simulink model "mdlWiW2025"  (R2024b)
settings: Solver=FixedStepAuto  StartTime=0.0  StopTime=p.simTime  FixedStep=5e-5  MaxStep=1e-4  RelTol=1e-3
values from neighbouring files (symbols this model uses):
  a0_WT_Act_DC_Inv = a0    [RunTestCasesWiW2025.m]    (also in mainWiW2025.m)
  A_WT_Act_DC_Inv = A    [RunTestCasesWiW2025.m]    (also in mainWiW2025.m)
  B_WT_Act_DC_Inv = Bu    [RunTestCasesWiW2025.m]    (also in mainWiW2025.m)
  Bd_WT_Act_DC_Inv = Bd    [RunTestCasesWiW2025.m]    (also in mainWiW2025.m)
  Cag = p.LTIAngleGen.Cz(1,:)    [RunTestCasesWiW2025.m]    (also in mainWiW2025.m)
  Cd_WT_Act_DC_Inv = Cd    [RunTestCasesWiW2025.m]    (also in mainWiW2025.m)
  Cu_WT_Act_DC_Inv = Cu    [RunTestCasesWiW2025.m]    (also in mainWiW2025.m)
  Cx_WT_Act_DC_Inv = Cx    [RunTestCasesWiW2025.m]    (also in mainWiW2025.m)
  p = loadTestCasesWiW2025(p)    [RunTestCasesWiW2025.m]    (also in mainWiW2025.m)
  parWT_Init = calcInitWTV2(parWT_Init,parWT,PrefInv0,v_wind_pu0)    [RunTestCasesWiW2025.m]    (also in mainWiW2025.m)
  xInit_WT_Act_DC_Inv = x0    [RunTestCasesWiW2025.m]    (also in mainWiW2025.m)
undefined symbols (not defined in the file or in its folder): DiscIntNeverNeededParam, height, KuDC, parDC, parInvLinMdl, parSim, parWT
libraries: simulink x14, simulink_extras x6
settings Model: Creator=jb  LastModifiedBy=jb

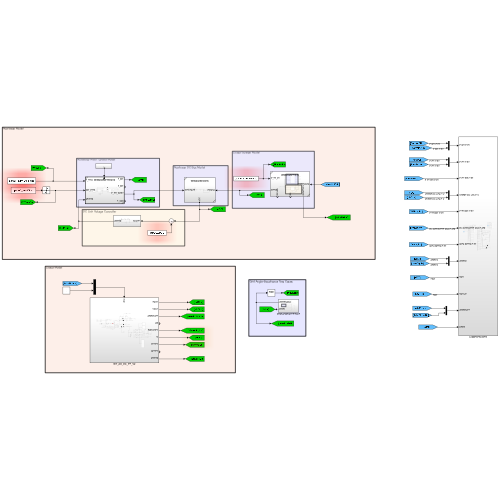
[thumbnail: Simulink's stored preview of the top-level diagram]
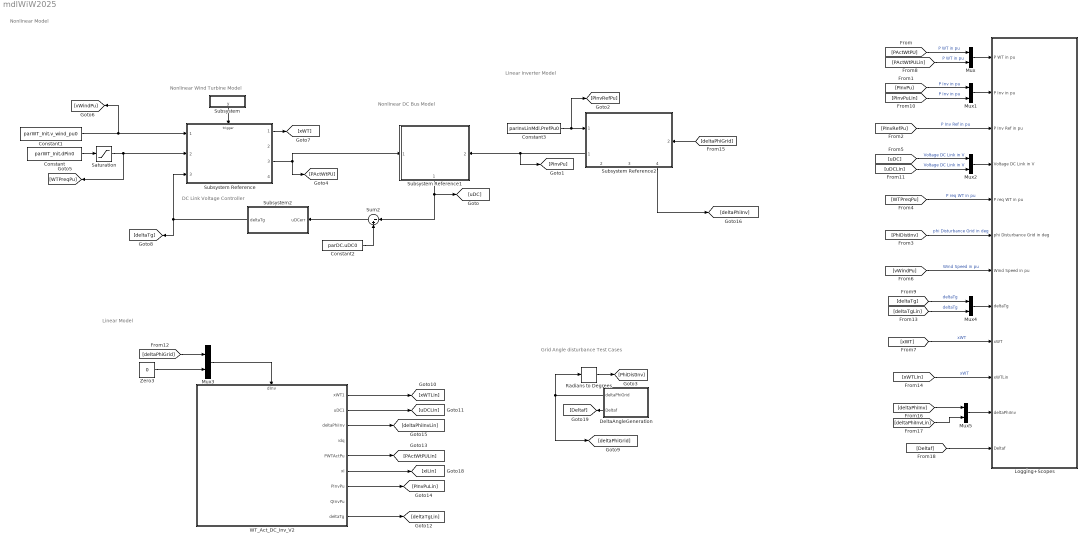
== system mdlWiW2025 ==
  note: Linear Model
  note: Nonlinear Model
  note: Grid Angle disturbance Test Cases
  note: Linear Inverter Model
  note: Nonlinear DC Bus Model
  note: Nonlinear Wind Turbine Model
  note: DC Link Voltage Controller
  Constant : Constant  Value=parWT_Init.dPin0
  Constant1 : Constant  Value=parWT_Init.v_wind_pu0
  Constant2 : Constant  Value=parDC.uDC0
  Constant3 : Constant  Value=parInvLinMdl.PrefPu0
  DeltaAngleGeneration : Subsystem
  Logging+Scopes : Subsystem
  Mux{,1..5} (6 alike) : Mux  Inputs=2
  Radians to Degrees : simulink_extras/Transformations/Radians to Degrees
  Saturation : Saturate  UpperLimit=1  LowerLimit=0
  Subsystem : Subsystem
      settings: PortSchema="{\"entries\":[{\"content\":{\"sides\":[{\"content\":{},\"type\":\"ConnectorPlacement.EquallySpacedRectSide\",\"uuid\":\"face2676-c510-409b-bee4-6c32a14faacb\"},{\"content\":{\"side\":\"RIGHT\"},\"type\":\"ConnectorPlacement.EquallySpacedRectSide\",\"uuid\":\"830bd05e-6053-45eb-9a2c-0b303f31509f\"},{\"content\":{\"side\":\"TOP\"},\"type\":\"ConnectorPlacement.EquallySpacedRectSide\",\"uuid\":\"8cce3491-981c-4252-b01c-3725d9c0f3f5\"},{\"content\":{\"connectorIds\":[\"Out1\"],\"side\":\"BOTTOM\"},\"type\":\"ConnectorPlacement.EquallySpacedRectSide\",\"uuid\":\"0505e35c-7957-4f95-90e0-2f2f2a48fa2e\"}]},\"type\":\"ConnectorPlacement.EquallySpacedConnector\",\"uuid\":\"a006b626-9c6b-4b47-b9fe-26644a837cf6\"}],\"packageUris\":[\"http://schema.mathworks.com/mf0/Connector/R2020b\"],\"version\":\"1.0\"}"
  Subsystem Reference : Subsystem  ReferencedSubsystem=WiW2025WTSubV2
  Subsystem Reference1 : Subsystem  ReferencedSubsystem=WiW2025DCSub
      settings: PortSchema="{\"entries\":[{\"content\":{\"sides\":[{\"content\":{\"connectorIds\":[\"In1\"]},\"type\":\"ConnectorPlacement.EquallySpacedRectSide\",\"uuid\":\"af152640-0aea-4f78-87a2-77a2b6d9cc3d\"},{\"content\":{\"connectorIds\":[\"In2\"],\"side\":\"RIGHT\"},\"type\":\"ConnectorPlacement.EquallySpacedRectSide\",\"uuid\":\"c02e3cac-108b-419e-ba46-7a5e2003643a\"},{\"content\":{\"side\":\"TOP\"},\"type\":\"ConnectorPlacement.EquallySpacedRectSide\",\"uuid\":\"91b439c3-63cc-4837-83b1-e86f1ef1a4a8\"},{\"content\":{\"connectorIds\":[\"Out1\"],\"side\":\"BOTTOM\"},\"type\":\"ConnectorPlacement.EquallySpacedRectSide\",\"uuid\":\"d1b53956-1662-4620-938c-5b6d0f97b7d8\"}]},\"type\":\"ConnectorPlacement.EquallySpacedConnector\",\"uuid\":\"de17c35b-190b-4b93-b08c-74ec9942f8f8\"}],\"packageUris\":[\"http://schema.mathworks.com/mf0/Connector/R2020b\"],\"version\":\"1.0\"}"
  Subsystem Reference2 : Subsystem  ReferencedSubsystem=WIW2025InvSub
      settings: PortSchema="{\"entries\":[{\"content\":{\"sides\":[{\"content\":{\"connectorIds\":[\"In1\",\"Out1\"]},\"type\":\"ConnectorPlacement.EquallySpacedRectSide\",\"uuid\":\"cb46f29d-b99f-4ee2-b312-1d4d79ed2caa\"},{\"content\":{\"connectorIds\":[\"In2\"],\"side\":\"RIGHT\"},\"type\":\"ConnectorPlacement.EquallySpacedRectSide\",\"uuid\":\"26f24ffb-094e-4bd5-ac8a-0db6a0458604\"},{\"content\":{\"side\":\"TOP\"},\"type\":\"ConnectorPlacement.EquallySpacedRectSide\",\"uuid\":\"c74ec33e-f362-4649-ae41-595cc258bb20\"},{\"content\":{\"connectorIds\":[\"Out2\",\"Out3\",\"Out4\"],\"side\":\"BOTTOM\"},\"type\":\"ConnectorPlacement.EquallySpacedRectSide\",\"uuid\":\"007ad1bf-c446-4ada-ae47-7c61a598a283\"}]},\"type\":\"ConnectorPlacement.EquallySpacedConnector\",\"uuid\":\"d7ac4c6f-570b-43ee-bac2-909fe494d4ed\"}],\"packageUris\":[\"http://schema.mathworks.com/mf0/Connector/R2020b\"],\"version\":\"1.0\"}"
  Subsystem2 : Subsystem
  Sum2 : Sum  Inputs=|-+
  WT_Act_DC_Inv_V2 : Subsystem
      settings: PortSchema="{\"entries\":[{\"content\":{\"sides\":[{\"content\":{},\"type\":\"ConnectorPlacement.EquallySpacedRectSide\",\"uuid\":\"d496482a-58bf-4391-9899-88596b85405c\"},{\"content\":{\"connectorIds\":[\"Out1\",\"Out2\",\"Out3\",\"Out4\",\"Out5\",\"Out6\",\"Out7\",\"Out8\",\"Out9\"],\"side\":\"RIGHT\"},\"type\":\"ConnectorPlacement.EquallySpacedRectSide\",\"uuid\":\"a3404192-e98c-40d4-9c55-e554f3dcbbe4\"},{\"content\":{\"connectorIds\":[\"In1\"],\"side\":\"TOP\"},\"type\":\"ConnectorPlacement.EquallySpacedRectSide\",\"uuid\":\"9344e298-d4d2-4a1e-a643-46297d368621\"}]},\"type\":\"ConnectorPlacement.EquallySpacedConnector\",\"uuid\":\"f7f68960-7837-437b-8e14-1803fee5da4e\"}],\"packageUris\":[\"http://schema.mathworks.com/mf0/Connector/R2020b\"],\"version\":\"1.0\"}"
  Zero3 : Constant  Value=0  OutDataTypeStr=Inherit: Inherit via back propagation
  wires:
  Constant/1 -> Saturation/1
  DeltaAngleGeneration/1(deltaPhiGrid) -> [deltaPhiGrid], Radians to Degrees/1
  Constant1/1 -> Subsystem Reference/1, [vWindPu]
  Radians to Degrees/1 -> [PhiDistInv]
  Saturation/1 -> Subsystem Reference/2, [WTPreqPu]
  Subsystem Reference/1 -> [xWT]
  Subsystem/1(y) -> Subsystem Reference/Trigger
  Sum2/1 -> Subsystem2/1(uDCerr)
  Constant2/1 -> Sum2/2
  Subsystem Reference1/1 -> Sum2/1, [uDC]
  Subsystem Reference/3 -> Subsystem Reference1/1, [PActWtPU]
  Subsystem2/1(deltaTg) -> [deltaTg], Subsystem Reference/3
  Constant3/1 -> [PInvRefPu], Subsystem Reference2/1
  Subsystem Reference2/1 -> [PInvPu], Subsystem Reference1/2
  [deltaPhiGrid] -> Mux3/1
  Mux3/1 -> WT_Act_DC_Inv_V2/1(dInv)
  Zero3/1 -> Mux3/2
  WT_Act_DC_Inv_V2/1(xWT1) -> [xWTLin]
  WT_Act_DC_Inv_V2/2(uDC1) -> [uDCLin]
  WT_Act_DC_Inv_V2/9(deltaTg) -> [deltaTgLin]
  WT_Act_DC_Inv_V2/7(PInvPu) -> [PInvPuLin]
  [PActWtPU] -> Mux/1  "P WT in pu"
  [PInvPu] -> Mux1/1  "P Inv in pu"
  [PInvRefPu] -> Logging+Scopes/3(P Inv Ref in pu)  "P Inv Ref in pu"
  [uDC] -> Mux2/1  "Voltage DC Link in V"
  [deltaTg] -> Mux4/1  "deltaTg"
  [xWT] -> Logging+Scopes/9(xWT)  "xWT"
  [vWindPu] -> Logging+Scopes/7(Wind Speed in pu)  "Wind Speed in pu"
  [PhiDistInv] -> Logging+Scopes/6(phi Disturbance Grid in deg)  "phi Disturbance Grid in deg"
  [WTPreqPu] -> Logging+Scopes/5(P req WT in pu)  "P req WT in pu"
  Mux2/1 -> Logging+Scopes/4(Voltage DC Link in V)
  Mux1/1 -> Logging+Scopes/2(P Inv in pu)
  Mux/1 -> Logging+Scopes/1(P WT in pu)
  [PActWtPULin] -> Mux/2  "P WT in pu"
  [PInvPuLin] -> Mux1/2  "P Inv in pu"
  [uDCLin] -> Mux2/2  "Voltage DC Link in V"
  [deltaTgLin] -> Mux4/2  "deltaTg"
  Mux4/1 -> Logging+Scopes/8(deltaTg)
  [xWTLin] -> Logging+Scopes/10(xWTLin)  "xWT"
  [deltaPhiGrid] -> Subsystem Reference2/2
  WT_Act_DC_Inv_V2/5(PWTActPu) -> [PActWtPULin]
  WT_Act_DC_Inv_V2/3(deltaPhiInv) -> [deltaPhiInvLin]
  Subsystem Reference2/4 -> [deltaPhiInv]
  Mux5/1 -> Logging+Scopes/11(deltaPhiInv)
  [deltaPhiInv] -> Mux5/1
  [deltaPhiInvLin] -> Mux5/2
  WT_Act_DC_Inv_V2/6(xI) -> [xILin]
  DeltaAngleGeneration/2(Deltaf) -> [Deltaf]
  [Deltaf] -> Logging+Scopes/12(Deltaf)

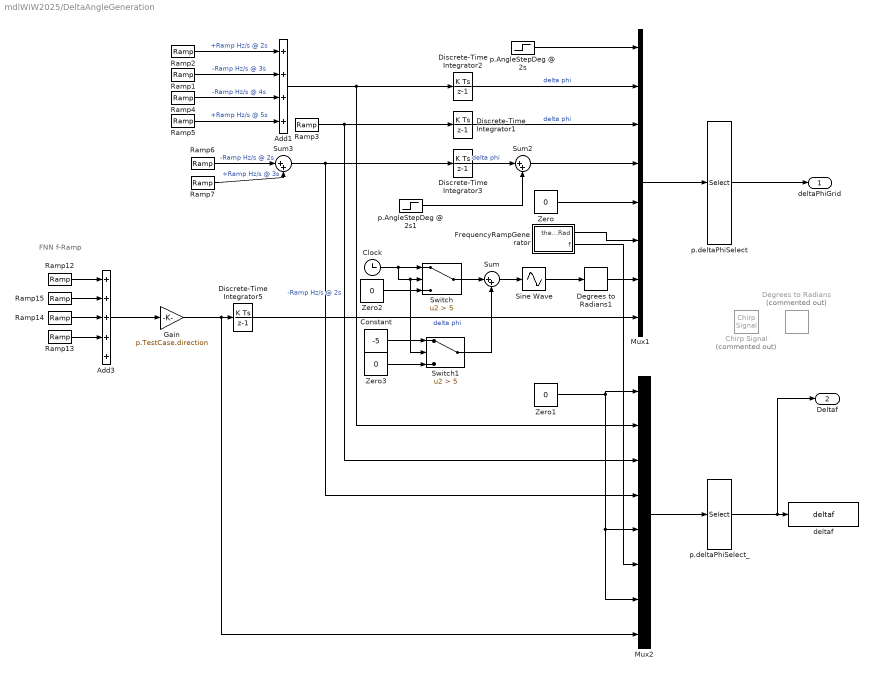
== system mdlWiW2025/DeltaAngleGeneration ==
  note: FNN f-Ramp
  Add1 : Sum  Inputs=++++
  Add3 : Sum  Inputs=+++++
  Chirp Signal : simulink/Sources/Chirp Signal  Commented=on  f1=0.1  T=80  f2=5
  Clock : Clock
  Constant : Constant  Value=-5
  Degrees to Radians : simulink_extras/Transformations/Degrees to Radians  Commented=on
  Degrees to Radians1 : simulink_extras/Transformations/Degrees to Radians
  Discrete-Time Integrator{1..3,5} (4 alike) : DiscreteIntegrator  SampleTime=-1  ICPrevOutput=DiscIntNeverNeededParam  ICPrevScaledInput=DiscIntNeverNeededParam
  FrequencyRampGenerator : Subsystem
  Gain : Gain  Gain=p.TestCase.direction
  Mux1 : Mux  Inputs=8
  Mux2 : Mux  Inputs=8
  Ramp1 : simulink/Sources/Ramp  slope=-p.FrequencyRamp  start=3  InitialOutput=0
  Ramp12 : simulink/Sources/Ramp  slope=-2  start=p.TestCase.t0  InitialOutput=0
  Ramp13 : simulink/Sources/Ramp  slope=-1  start=p.TestCase.t0+4  InitialOutput=0
  Ramp14 : simulink/Sources/Ramp  slope=+1/3+1  start=p.TestCase.t0+2.5  InitialOutput=0
  Ramp15 : simulink/Sources/Ramp  slope=+2-1/3  start=p.TestCase.t0+1  InitialOutput=0
  Ramp2 : simulink/Sources/Ramp  slope=p.FrequencyRamp  start=2  InitialOutput=0
  Ramp3 : simulink/Sources/Ramp  slope=-p.FrequencyRamp  start=2  InitialOutput=0
  Ramp4 : simulink/Sources/Ramp  slope=-p.FrequencyRamp  start=4  InitialOutput=0
  Ramp5 : simulink/Sources/Ramp  slope=p.FrequencyRamp  start=5  InitialOutput=0
  Ramp6 : simulink/Sources/Ramp  slope=-p.FrequencyRamp  start=2  InitialOutput=0
  Ramp7 : simulink/Sources/Ramp  slope=p.FrequencyRamp  start=3  InitialOutput=0
  Sine Wave : Sin  TimeSource=Use external signal  Amplitude=p.AmplitudeSineInput  Frequency=p.FrequencySineInput*pi*2  SampleTime=0
  Sum : Sum  Inputs=|++
  Sum2 : Sum  Inputs=|++
  Sum3 : Sum  Inputs=|++
  Switch : Switch  Criteria=u2 > Threshold  Threshold=5  SaturateOnIntegerOverflow=off  InputSameDT=off
  Switch1 : Switch  Criteria=u2 > Threshold  Threshold=5  SaturateOnIntegerOverflow=off  InputSameDT=off
  Zero{,1..3} (4 alike) : Constant  Value=0  OutDataTypeStr=Inherit: Inherit via back propagation
  deltaf : ToWorkspace  VariableName=deltaf  SaveFormat=Structure With Time  SampleTime=-1
  p.AngleStepDeg @ 2s : Step  Time=2  After=deg2rad(p.AngleStepDeg)  SampleTime=0
  p.AngleStepDeg @ 2s1 : Step  Time=2  After=deg2rad(p.AngleStepDeg)  SampleTime=0
  p.deltaPhiSelect : Selector  InputPortWidth=8  IndexOptions=Index vector (dialog)  Indices=[p.deltaPhiSelect]  OutputSizes=1
  p.deltaPhiSelect_ : Selector  InputPortWidth=8  IndexOptions=Index vector (dialog)  Indices=[p.deltaPhiSelect]  OutputSizes=1
  deltaPhiGrid : Outport
  Deltaf : Outport  Port=2
  wires:
  Ramp7/1 -> Sum3/2  "+Ramp Hz/s @ 3s"
  Ramp5/1 -> Add1/4  "+Ramp Hz/s @ 5s"
  p.AngleStepDeg @ 2s/1 -> Mux1/1
  Sum3/1 -> Discrete-Time Integrator3/1, Mux2/4
  Discrete-Time Integrator2/1 -> Mux1/2  "delta phi"
  Mux1/1 -> p.deltaPhiSelect/1
  p.deltaPhiSelect/1 -> deltaPhiGrid/1
  Ramp2/1 -> Add1/1  "+Ramp Hz/s @ 2s"
  Discrete-Time Integrator1/1 -> Mux1/3  "delta phi"
  Sum2/1 -> Mux1/4
  Ramp6/1 -> Sum3/1  "-Ramp Hz/s @ 2s"
  Ramp3/1 -> Discrete-Time Integrator1/1, Mux2/3  "-Ramp Hz/s @ 2s"
  p.AngleStepDeg @ 2s1/1 -> Sum2/2
  Zero/1 -> Mux1/5
  Ramp4/1 -> Add1/3  "-Ramp Hz/s @ 4s"
  Discrete-Time Integrator3/1 -> Sum2/1  "delta phi"
  Ramp1/1 -> Add1/2  "-Ramp Hz/s @ 3s"
  Add1/1 -> Discrete-Time Integrator2/1, Mux2/2
  Degrees to Radians1/1 -> Mux1/7
  Mux2/1 -> p.deltaPhiSelect_/1
  Zero1/1 -> Mux2/1, Mux2/7, Mux2/5
  p.deltaPhiSelect_/1 -> Deltaf/1, deltaf/1
  Gain/1 -> Mux2/8, Discrete-Time Integrator5/1
  Add3/1 -> Gain/1
  Discrete-Time Integrator5/1 -> Mux1/8  "delta phi"
  Ramp13/1 -> Add3/4
  Ramp14/1 -> Add3/3
  Ramp12/1 -> Add3/1
  Ramp15/1 -> Add3/2
  Clock/1 -> Switch1/2, Switch/2, Switch/1
  Zero2/1 -> Switch/3
  Sine Wave/1 -> Degrees to Radians1/1
  Zero3/1 -> Switch1/3
  Constant/1 -> Switch1/1
  Sum/1 -> Sine Wave/1
  Switch/1 -> Sum/1
  Switch1/1 -> Sum/2
  FrequencyRampGenerator/1(thetaRad) -> Mux1/6
  FrequencyRampGenerator/2(f) -> Mux2/6

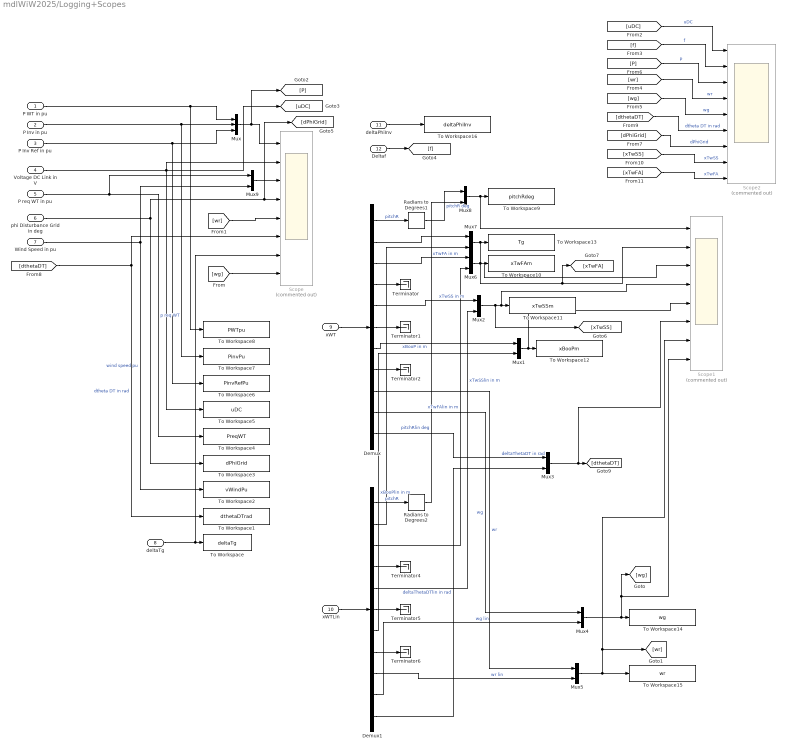
== system mdlWiW2025/Logging+Scopes ==
  P WT in pu : Inport
  P Inv in pu : Inport  Port=2
  P Inv Ref in pu : Inport  Port=3
  Voltage DC Link in V : Inport  Port=4
  P req WT in pu : Inport  Port=5
  phi Disturbance Grid in deg : Inport  Port=6
  Wind Speed in pu : Inport  Port=7
  deltaTg : Inport  Port=8
  xWT : Inport  Port=9
  xWTLin : Inport  Port=10
  deltaPhiInv : Inport  Port=11
  Deltaf : Inport  Port=12
  Demux : Demux  Outputs=11
  Demux1 : Demux  Outputs=11
  Mux : Mux  Inputs=3
  Mux{1..9} (9 alike) : Mux  Inputs=2
  Radians to Degrees1 : simulink_extras/Transformations/Radians to Degrees
  Radians to Degrees2 : simulink_extras/Transformations/Radians to Degrees
  Scope : Scope  Commented=on  NumInputPorts=8
  Scope1 : Scope  Commented=on  NumInputPorts=8
  Scope2 : Scope  Commented=on  NumInputPorts=9
  Terminator{,1..2,4..6} (6 alike) : Terminator
  To Workspace : ToWorkspace  VariableName=deltaTg  SaveFormat=Structure With Time  SampleTime=-1
  To Workspace1 : ToWorkspace  VariableName=dthetaDTrad  SaveFormat=Structure With Time  SampleTime=-1
  To Workspace10 : ToWorkspace  VariableName=xTwFAm  SaveFormat=Structure With Time  SampleTime=-1
  To Workspace11 : ToWorkspace  VariableName=xTwSSm  SaveFormat=Structure With Time  SampleTime=-1
  To Workspace12 : ToWorkspace  VariableName=xBooPm  SaveFormat=Structure With Time  SampleTime=-1
  To Workspace13 : ToWorkspace  VariableName=Tg  SaveFormat=Structure With Time  SampleTime=-1
  To Workspace14 : ToWorkspace  VariableName=wg  SaveFormat=Structure With Time  SampleTime=-1
  To Workspace15 : ToWorkspace  VariableName=wr  SaveFormat=Structure With Time  SampleTime=-1
  To Workspace16 : ToWorkspace  VariableName=deltaPhiInv  SaveFormat=Structure With Time  SampleTime=-1
  To Workspace2 : ToWorkspace  VariableName=vWindPu  SaveFormat=Structure With Time  SampleTime=-1
  To Workspace3 : ToWorkspace  VariableName=dPhiGrid  SaveFormat=Structure With Time  SampleTime=-1
  To Workspace4 : ToWorkspace  VariableName=PreqWT  SaveFormat=Structure With Time  SampleTime=-1
  To Workspace5 : ToWorkspace  VariableName=uDC  SaveFormat=Structure With Time  SampleTime=-1
  To Workspace6 : ToWorkspace  VariableName=PinvRefPu  SaveFormat=Structure With Time  SampleTime=-1
  To Workspace7 : ToWorkspace  VariableName=PinvPu  SaveFormat=Structure With Time  SampleTime=-1
  To Workspace8 : ToWorkspace  VariableName=PWTpu  SaveFormat=Structure With Time  SampleTime=-1
  To Workspace9 : ToWorkspace  VariableName=pitchRdeg  SaveFormat=Structure With Time  SampleTime=-1
  wires:
  P Inv in pu/1 -> Mux/2, To Workspace7/1
  Demux/6 -> Terminator1/1
  P req WT in pu/1 -> Mux9/1, To Workspace4/1  "p req WT"
  xWT/1 -> Demux/1
  Demux/4 -> Terminator/1
  Voltage DC Link in V/1 -> Scope/2, To Workspace5/1, [uDC]
  Mux/1 -> [P], Scope/1
  Demux/1 -> Radians to Degrees1/1  "pitchR"
  Demux/8 -> Terminator2/1
  P WT in pu/1 -> Mux/1, To Workspace8/1
  Wind Speed in pu/1 -> Mux9/2, To Workspace2/1  "wind speed pu"
  phi Disturbance Grid in deg/1 -> Scope/4, [dPhiGrid], To Workspace3/1
  P Inv Ref in pu/1 -> Mux/3, To Workspace6/1
  Demux/11 -> Mux3/1  "deltaThetaDT in rad"
  [dthetaDT] -> Scope/6, To Workspace1/1  "dtheta DT in rad"
  deltaTg/1 -> Scope/7, To Workspace/1
  Demux/9 -> Mux5/1  "wr"
  Demux/10 -> Mux4/1  "wg"
  Demux1/1 -> Radians to Degrees2/1  "pitchR"
  Demux1/11 -> Mux3/2  "deltaThetaDTlin in rad"
  Demux1/6 -> Terminator5/1
  Demux1/7 -> Mux1/2  "xBooPlin in m"
  xWTLin/1 -> Demux1/1
  Demux1/8 -> Terminator6/1
  Demux1/4 -> Terminator4/1
  Mux3/1 -> Scope1/6, [dthetaDT]
  Mux4/1 -> [wg], Scope1/8, To Workspace14/1
  Demux1/10 -> Mux4/2  "wg lin"
  Demux1/9 -> Mux5/2  "wr lin"
  deltaPhiInv/1 -> To Workspace16/1
  Mux5/1 -> [wr], Scope1/7, To Workspace15/1
  Mux1/1 -> Scope1/5, To Workspace12/1
  Demux/7 -> Mux1/1  "xBooP in m"
  Mux2/1 -> [xTwSS], Scope1/4, To Workspace11/1
  Demux/5 -> Mux2/1  "xTwSS in m"
  Demux1/5 -> Mux2/2  "xTwSSlin in m"
  Mux6/1 -> Scope1/3, To Workspace10/1
  Demux1/3 -> Mux6/2  "xTwFAlin in m"
  Demux/3 -> Mux6/1  "xTwFA in m"
  Mux7/1 -> [xTwFA], Scope1/2, To Workspace13/1
  Demux/2 -> Mux7/1
  Demux1/2 -> Mux7/2
  Mux8/1 -> Scope1/1, To Workspace9/1
  Radians to Degrees1/1 -> Mux8/1  "pitchR deg"
  Radians to Degrees2/1 -> Mux8/2  "pitchRlin deg"
  [wg] -> Scope/8
  Mux9/1 -> Scope/3
  [wr] -> Scope/5
  Deltaf/1 -> [f]
  [uDC] -> Scope2/1  "uDC"
  [f] -> Scope2/2  "f"
  [P] -> Scope2/3  "P"
  [wr] -> Scope2/4  "wr"
  [wg] -> Scope2/5  "wg"
  [dthetaDT] -> Scope2/6  "dtheta DT in rad"
  [dPhiGrid] -> Scope2/7  "dPhiGrid"
  [xTwSS] -> Scope2/8  "xTwSS"
  [xTwFA] -> Scope2/9  "xTwFA"

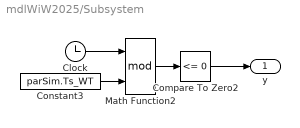
== system mdlWiW2025/Subsystem ==
  Clock : Clock
  Compare To Zero2 : simulink/Logic and Bit Operations/Compare To Zero  relop=<=  OutDataTypeStr=boolean
  Constant3 : Constant  Value=parSim.Ts_WT
  Math Function2 : Math  Operator=mod
  y : Outport
  wires:
  Clock/1 -> Math Function2/1
  Constant3/1 -> Math Function2/2
  Math Function2/1 -> Compare To Zero2/1
  Compare To Zero2/1 -> y/1

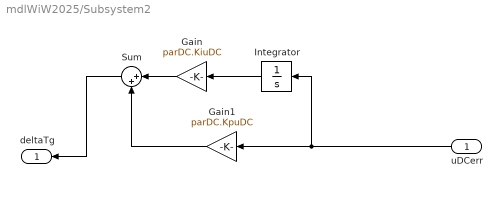
== system mdlWiW2025/Subsystem2 ==
  uDCerr : Inport
  Gain : Gain  Gain=parDC.KiuDC
  Gain1 : Gain  Gain=parDC.KpuDC
  Integrator : Integrator
  Sum : Sum  Inputs=|++
  deltaTg : Outport
  wires:
  uDCerr/1 -> Integrator/1, Gain1/1
  Integrator/1 -> Gain/1
  Gain/1 -> Sum/1
  Gain1/1 -> Sum/2
  Sum/1 -> deltaTg/1

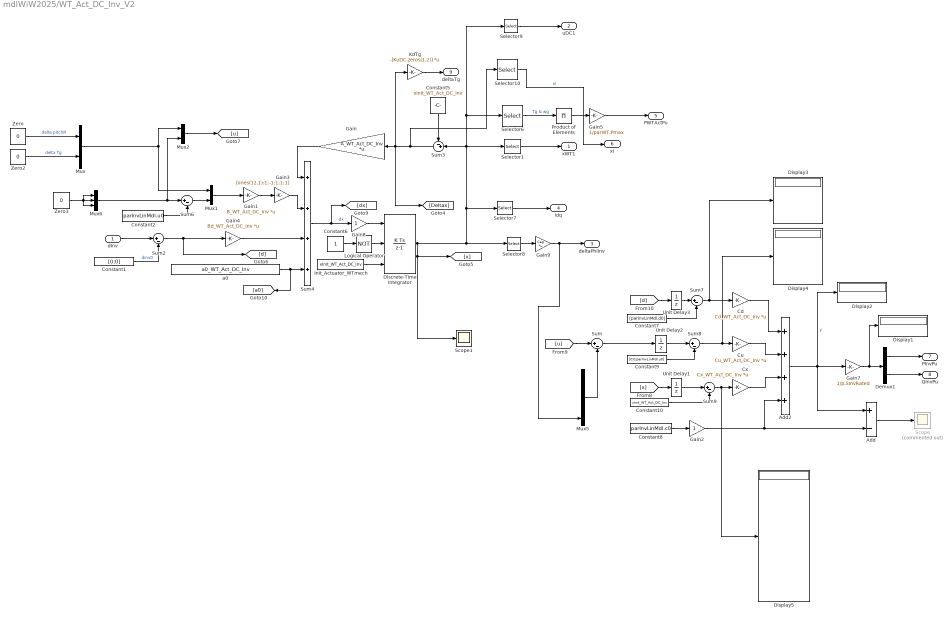
== system mdlWiW2025/WT_Act_DC_Inv_V2 ==
  dInv : Inport
  Add : Sum  Inputs=+-
  Add2 : Sum  Inputs=++++
  Cd : Gain  Gain=Cd_WT_Act_DC_Inv  Multiplication=Matrix(K*u)
  Constant1 : Constant  Value=[0;0]
  Constant10 : Constant  Value=xInit_WT_Act_DC_Inv
  Constant2 : Constant  Value=parInvLinMdl.u0
  Constant5 : Constant  Value=xInit_WT_Act_DC_Inv
  Constant6 : Constant
  Constant7 : Constant  Value=[parInvLinMdl.d0]
  Constant8 : Constant  Value=parInvLinMdl.c0
  Constant9 : Constant  Value=[0;0;parInvLinMdl.u0]
  Cu : Gain  Gain=Cu_WT_Act_DC_Inv  Multiplication=Matrix(K*u)
  Cx : Gain  Gain=Cx_WT_Act_DC_Inv  Multiplication=Matrix(K*u)
  Demux1 : Demux  Outputs=2
  Discrete-Time Integrator : DiscreteIntegrator  ExternalReset=level  InitialConditionSource=external  SampleTime=-1  ICPrevOutput=DiscIntNeverNeededParam  ICPrevScaledInput=DiscIntNeverNeededParam
  Display{1..5} (5 alike) : Display
  Gain : Gain  Gain=A_WT_Act_DC_Inv  Multiplication=Matrix(K*u)
  Gain1 : Gain  Gain=B_WT_Act_DC_Inv  Multiplication=Matrix(K*u)
  Gain2 : Gain
  Gain3 : Gain  Gain=[ones(12,1);1;-1;1;1;1]
  Gain4 : Gain  Gain=Bd_WT_Act_DC_Inv  Multiplication=Matrix(K*u)
  Gain5 : Gain  Gain=1/parWT.Pmax
  Gain7 : Gain  Gain=1/p.SInvRated
  Gain8 : Gain
  Gain9 : Gain  Gain=Cag  Multiplication=Matrix(K*u)
  Init_Actuator_WTmech : Constant  Value=xInit_WT_Act_DC_Inv  VectorParams1D=off
  KdTg : Gain  Gain=-[KuDC,zeros(1,2)]  Multiplication=Matrix(K*u)
  Logical Operator : Logic  Operator=NOT  AllPortsSameDT=off  OutDataTypeStr=boolean
  Mux : Mux  Inputs=2
  Mux1 : Mux  Inputs=2
  Mux2 : Mux  Inputs=2
  Mux5 : Mux  Inputs=5
  Mux6 : Mux  Inputs=3
  Product of Elements : Product  Inputs=*
  Scope : Scope  Commented=on
  Scope1 : Scope
  Selector1 : Selector  InputPortWidth=height(A_WT_Act_DC_Inv)  IndexOptions=Index vector (dialog)  Indices=[1:11]  OutputSizes=1
  Selector10 : Selector  InputPortWidth=height(A_WT_Act_DC_Inv)  IndexOptions=Index vector (dialog)  Indices=[12]  OutputSizes=1
  Selector6 : Selector  InputPortWidth=height(A_WT_Act_DC_Inv)  IndexOptions=Index vector (dialog)  Indices=[2,10]  OutputSizes=1
  Selector7 : Selector  InputPortWidth=height(A_WT_Act_DC_Inv)  IndexOptions=Index vector (dialog)  Indices=[13:14]  OutputSizes=1
  Selector8 : Selector  InputPortWidth=height(A_WT_Act_DC_Inv)  IndexOptions=Index vector (dialog)  Indices=[16:17]  OutputSizes=1
  Selector9 : Selector  InputPortWidth=height(A_WT_Act_DC_Inv)  IndexOptions=Index vector (dialog)  Indices=[12]  OutputSizes=1
  Sum{,2,6..9} (6 alike) : Sum  Inputs=|+-
  Sum3 : Sum  Inputs=-+|
  Sum4 : Sum  Inputs=++++
  Unit Delay1 : UnitDelay  SampleTime=-1  HasFrameUpgradeWarning=on
  Unit Delay2 : UnitDelay  SampleTime=-1  HasFrameUpgradeWarning=on
  Unit Delay3 : UnitDelay  SampleTime=-1  HasFrameUpgradeWarning=on
  Zero : Constant  Value=0  OutDataTypeStr=Inherit: Inherit via back propagation
  Zero2 : Constant  Value=0  OutDataTypeStr=Inherit: Inherit via back propagation
  Zero3 : Constant  Value=0  OutDataTypeStr=Inherit: Inherit via back propagation
  a0 : Constant  Value=a0_WT_Act_DC_Inv
  xWT1 : Outport
  uDC1 : Outport  Port=2
  deltaPhiInv : Outport  Port=3
  idq : Outport  Port=4
  PWTActPu : Outport  Port=5
  xI : Outport  Port=6
  PInvPu : Outport  Port=7
  QInvPu : Outport  Port=8
  deltaTg : Outport  Port=9
  wires:
  Constant5/1 -> Sum3/1
  Logical Operator/1 -> Discrete-Time Integrator/2
  Gain4/1 -> Sum4/3
  Sum4/1 -> [dx], Gain8/1  "dx"
  Init_Actuator_WTmech/1 -> Discrete-Time Integrator/3
  Constant6/1 -> Logical Operator/1
  Gain1/1 -> Gain3/1
  Zero/1 -> Mux/1  "delta pitchR"
  Gain/1 -> Sum4/1
  Mux/1 -> Mux1/1, Mux2/1
  Sum2/1 -> Gain4/1, [d]
  dInv/1 -> Sum2/1
  Constant1/1 -> Sum2/2  "dinv0"
  Zero2/1 -> Mux/2  "delta Tg"
  Sum6/1 -> Mux1/2
  Mux6/1 -> Sum6/1, Mux2/2
  Constant2/1 -> Sum6/2
  Gain3/1 -> Sum4/2
  a0/1 -> Sum4/4, [a0]
  Sum7/1 -> Cd/1, Display3/1
  Sum9/1 -> Display5/1, Cx/1
  Cu/1 -> Add2/2
  Add2/1 -> Gain7/1, Display2/1, Add/1  "y"
  Constant10/1 -> Sum9/2
  [x] -> Unit Delay1/1
  Demux1/2 -> QInvPu/1
  Cx/1 -> Add2/3
  Constant7/1 -> Sum7/2
  Cd/1 -> Add2/1
  Sum8/1 -> Display4/1, Cu/1
  Constant8/1 -> Gain2/1
  Gain7/1 -> Demux1/1, Display1/1
  Demux1/1 -> PInvPu/1
  [d] -> Unit Delay3/1
  Gain8/1 -> Discrete-Time Integrator/1
  Mux1/1 -> Gain1/1
  Unit Delay1/1 -> Sum9/1
  Unit Delay2/1 -> Sum8/1
  Unit Delay3/1 -> Sum7/1
  Constant9/1 -> Sum8/2
  Mux2/1 -> [u]
  Add/1 -> Scope/1
  Gain2/1 -> Add/2, Add2/4
  [u] -> Sum/1
  Sum/1 -> Unit Delay2/1
  Mux5/1 -> Sum/2
  Zero3/1 -> Mux6/1, Mux6/3, Mux6/2
  Selector10/1 -> xI/1  "xI"
  Selector9/1 -> uDC1/1
  Discrete-Time Integrator/1 -> [x], Scope1/1, Selector8/1, Selector7/1, Selector1/1, Selector6/1, Selector9/1, Sum3/2
  Selector1/1 -> xWT1/1
  Selector6/1 -> Product of Elements/1  "Tg & wg"
  Gain5/1 -> PWTActPu/1
  Selector7/1 -> idq/1
  Selector8/1 -> Gain9/1
  Gain9/1 -> Mux5/5, deltaPhiInv/1
  Product of Elements/1 -> Gain5/1
  KdTg/1 -> deltaTg/1
  Sum3/1 -> Selector10/1, KdTg/1, Gain/1, [Deltax]

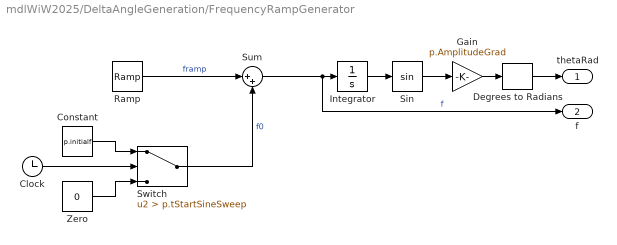
== system mdlWiW2025/DeltaAngleGeneration/FrequencyRampGenerator ==
  Clock : Clock
  Constant : Constant  Value=p.initialf
  Degrees to Radians : simulink_extras/Transformations/Degrees to Radians
  Gain : Gain  Gain=p.AmplitudeGrad
  Integrator : Integrator
  Ramp : simulink/Sources/Ramp  slope=p.targetfOfRamp/p.RampTime  start=p.tStartSineSweep  InitialOutput=0
  Sin : Trigonometry
  Sum : Sum  Inputs=|++
  Switch : Switch  Criteria=u2 > Threshold  Threshold=p.tStartSineSweep  SaturateOnIntegerOverflow=off  InputSameDT=off
  Zero : Constant  Value=0  OutDataTypeStr=Inherit: Inherit via back propagation
  thetaRad : Outport
  f : Outport  Port=2
  wires:
  Zero/1 -> Switch/3
  Sin/1 -> Gain/1
  Switch/1 -> Sum/2  "f0"
  Constant/1 -> Switch/1
  Integrator/1 -> Sin/1
  Ramp/1 -> Sum/1  "framp"
  Clock/1 -> Switch/2
  Sum/1 -> f/1, Integrator/1  "f"
  Degrees to Radians/1 -> thetaRad/1
  Gain/1 -> Degrees to Radians/1
